simulink model "test_4ph_core_coupling"  (R2018b)
settings: Solver=VariableStepAuto  StartTime=0.0  StopTime=10.0  RelTol=1e-3
undefined symbols (not defined in the file): Four, Phase
libraries: powerlib x5, typhoonHILlib x1
settings Model: Creator=Marcos  LastModifiedBy=USER
settings SFSimCC: SimUseLocalCustomCode=off
settings RTWCC: RTWUseLocalCustomCode=off

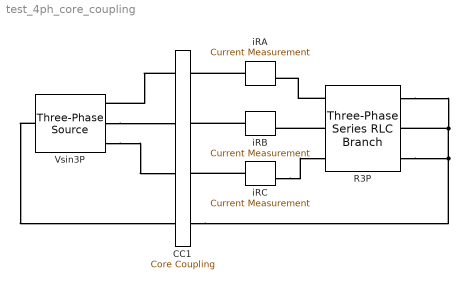
== system test_4ph_core_coupling ==
  CC1 : typhoonHILlib/Core Coupling  CouplingPhases=Four-Phase  IsTLM=off  snb_type_i=None  R1=100e3  C1=1e-6  fixed_snb_i=off  snb_type_v=None  R2=100e3  L1=1e-3  fixed_snb_v=off  CouplingType=Inductive  coup_cap=1e-3  coup_ind=1e-3  toggle_init=on  model_loaded=off  old_pat=typhoonPatterns/4P CC  old_size=15,196
      settings: SourceProductName=Typhoon HIL
  R3P : powerlib/Elements/Three-Phase Series RLC Branch  LConnTagsString=A|B|C  RConnTagsString=A|B|C  BranchType=R  Resistance=10  Inductance=1e-3  Capacitance=1e-6  Measurements=None
      settings: SourceProductName=Simscape Electrical
  Vsin3P : powerlib/Electrical Sources/Three-Phase Source  InternalConnection=Yn  VoltagePhases=off  Voltage=381  PhaseAngle=0  Voltage_phases=[25e3 25e3 25e3]/sqrt(3)  PhaseAngles_phases=[0 -120 +120]  Frequency=50  NonIdealSource=off  SpecifyImpedance=off  Resistance=0.8929  Inductance=16.58e-3  ShortCircuitLevel=100e6  BaseVoltage=25e3  XRratio=7  BusType=swing  Pref=10e3  Qref=0  Prefabc=[10e3, 10e3, 10e3]  Qrefabc=[0, 0, 0]  Qmin=-inf  Qmax=inf
      settings: SourceProductName=Simscape Electrical
  iRA : powerlib/Measurements/Current Measurement  PhasorSimulation=off  OutputType=Complex  PSBequivalent=0
      settings: SourceProductName=Simscape Electrical
  iRB : powerlib/Measurements/Current Measurement  PhasorSimulation=off  OutputType=Complex  PSBequivalent=0
      settings: SourceProductName=Simscape Electrical
  iRC : powerlib/Measurements/Current Measurement  PhasorSimulation=off  OutputType=Complex  PSBequivalent=0
      settings: SourceProductName=Simscape Electrical
  connections:
  CC1/LConn1 -- Vsin3P/RConn1
  R3P/LConn1 -- iRA/RConn1
  iRA/LConn1 -- CC1/RConn1
  R3P/LConn2 -- iRB/RConn1
  iRC/RConn1 -- R3P/LConn3
  R3P/RConn3 -- R3P/RConn2 -- R3P/RConn1 -- CC1/RConn4
  iRB/LConn1 -- CC1/RConn2
  iRC/LConn1 -- CC1/RConn3
  Vsin3P/RConn2 -- CC1/LConn2
  Vsin3P/RConn3 -- CC1/LConn3
  Vsin3P/LConn1 -- CC1/LConn4
